simulink model "comparetozero_complex_test"  (Simulink 8.4)
settings: Solver=ode45  StartTime=0.0  StopTime=10.0  RelTol=1e-3
libraries: simulink x2
settings Model: Creator=arnaud  LastModifiedBy=arnaud
settings DataIOCC: SaveFormat=Structure  SignalLoggingSaveFormat=Dataset
settings OptimizationCC: ExpressionDepthLimit=128
settings DebuggingCC: UnderspecifiedInitializationDetection=Simplified  MergeDetectMultiDrivingBlocksExec=error  FcnCallInpInsideContextMsg=EnableAllAsError  StateNameClashWarn=none
settings GRTTargetCC: CombineOutputUpdateFcns=on  GRTInterface=off

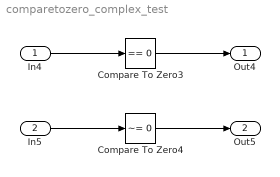
== system comparetozero_complex_test ==
  In4 : Inport  OutDataTypeStr=double  PortDimensions=3
      settings: SignalType=complex
  In5 : Inport  Port=2  OutDataTypeStr=int8  PortDimensions=3
      settings: SignalType=complex
  Compare To Zero3 : simulink/Logic and Bit Operations/Compare To Zero  relop===  OutDataTypeStr=boolean
  Compare To Zero4 : simulink/Logic and Bit Operations/Compare To Zero  relop=~=  OutDataTypeStr=boolean
  Out4 : Outport
  Out5 : Outport  Port=2
  wires:
  Compare To Zero3/1 -> Out4/1
  In4/1 -> Compare To Zero3/1
  Compare To Zero4/1 -> Out5/1
  In5/1 -> Compare To Zero4/1
